simulink model "SOH_RLS_estimator_prev"  (R2024a)
settings: configuration reference "BMS_Base_ModelReferencingConfig" (kept outside this file)
values from neighbouring files (symbols this model uses):
  BATTERY_MODULE_CAPACITY_AH = 51.0    [ParametersDataDictionary.sldd]    (also in SOXDictionary.sldd; SOXDictionaryGotion.sldd = 116.0
  SOH_DOD_THRESHOLD = 0.1    [SOXDictionary.sldd]    (also in SOXDictionaryGotion.sldd = 0.1
  SOH_ESTIM_INIT = 1.0    [SOXDictionary.sldd]    (also in SOXDictionaryGotion.sldd = 1.0
  SOH_INITIAL_COVARIANCE = 1.0    [SOXDictionary.sldd]    (also in SOXDictionaryGotion.sldd = 1.0
  SOH_LAMBDA = 0.9995    [SOXDictionary.sldd]    (also in SOXDictionaryGotion.sldd = 0.9995
  SOH_TIMESTEP = 1.0    [SOXDictionary.sldd]    (also in SOXDictionaryGotion.sldd = 1.0
  TOTAL_N_CELL_VOLTAGE = 24    [SOXDictionary.sldd]
settings Model: DataDictionary=BcuModel.sldd  SimulationMode=accelerator  Creator=mmackenzie  LastModifiedBy=jgavidia
settings ConfigSetRef: SourceName=BMS_Base_ModelReferencingConfig

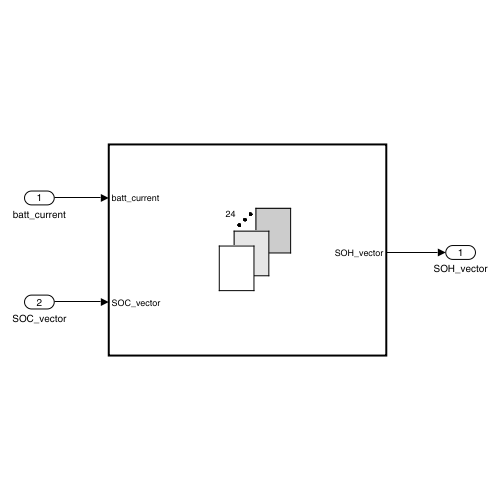
[thumbnail: Simulink's stored preview of the top-level diagram]
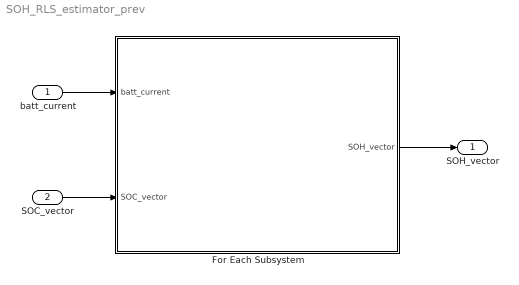
== system SOH_RLS_estimator_prev ==
  batt_current : Inport  OutDataTypeStr=int32  PortDimensions=1
  SOC_vector : Inport  Port=2  OutDataTypeStr=uint16  PortDimensions=[TOTAL_N_CELL_VOLTAGE,1]
  For Each Subsystem : Subsystem  TreatAsAtomicUnit=on
  SOH_vector : Outport  OutDataTypeStr=single  PortDimensions=[TOTAL_N_CELL_VOLTAGE,1]
  wires:
  batt_current/1 -> For Each Subsystem/1(batt_current)
  SOC_vector/1 -> For Each Subsystem/2(SOC_vector)
  For Each Subsystem/1(SOH_vector) -> SOH_vector/1

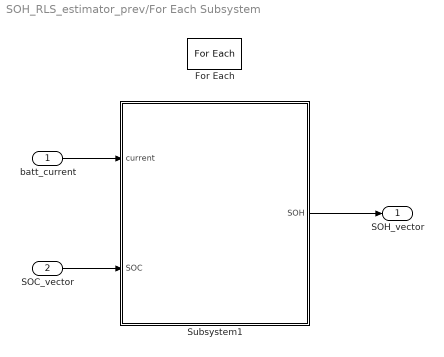
== system SOH_RLS_estimator_prev/For Each Subsystem ==
  batt_current : Inport  OutDataTypeStr=int32  PortDimensions=1
  SOC_vector : Inport  Port=2  OutDataTypeStr=uint16  PortDimensions=1  Partition=on  PartitionDimension=1  PartitionWidth=1  PartitionOffset=0
  For Each : ForEach  DisableCoverage=on
  Subsystem1 : Subsystem
  SOH_vector : Outport  OutDataTypeStr=single  PortDimensions=1  ConcatenationDimension=1
  wires:
  Subsystem1/1(SOH) -> SOH_vector/1
  batt_current/1 -> Subsystem1/1(current)
  SOC_vector/1 -> Subsystem1/2(SOC)

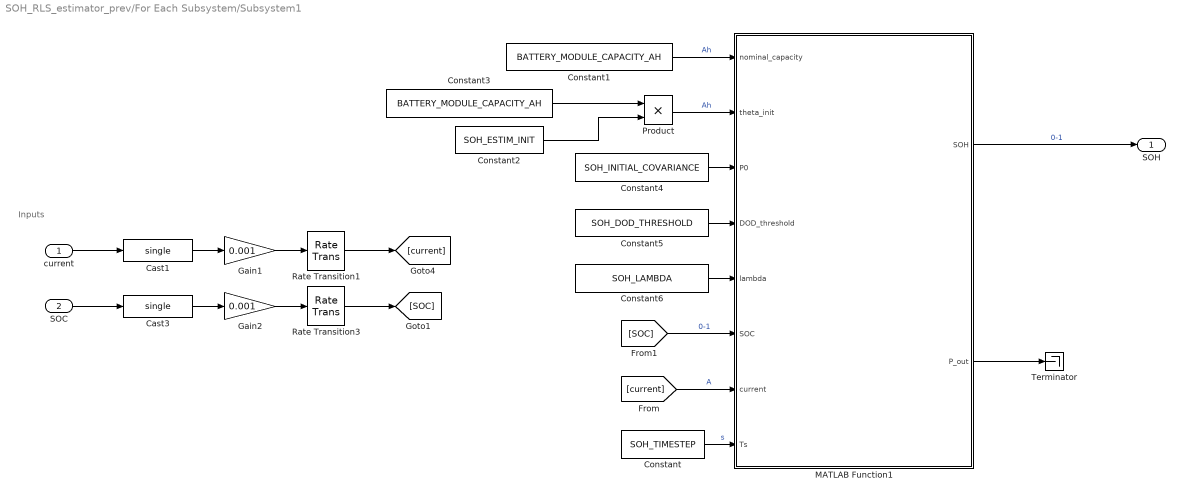
== system SOH_RLS_estimator_prev/For Each Subsystem/Subsystem1 ==
  note: Inputs
  current : Inport  OutDataTypeStr=int32  PortDimensions=1
  SOC : Inport  Port=2  OutDataTypeStr=uint16  PortDimensions=1
  Cast1 : DataTypeConversion  OutDataTypeStr=single  SaturateOnIntegerOverflow=off  RndMeth=Floor
  Cast3 : DataTypeConversion  OutDataTypeStr=single  SaturateOnIntegerOverflow=off  RndMeth=Floor
  Constant : Constant  Value=SOH_TIMESTEP
  Constant1 : Constant  Value=BATTERY_MODULE_CAPACITY_AH
  Constant2 : Constant  Value=SOH_ESTIM_INIT
  Constant3 : Constant  Value=BATTERY_MODULE_CAPACITY_AH
  Constant4 : Constant  Value=SOH_INITIAL_COVARIANCE
  Constant5 : Constant  Value=SOH_DOD_THRESHOLD
  Constant6 : Constant  Value=SOH_LAMBDA
  Gain1 : Gain  Gain=0.001
  Gain2 : Gain  Gain=0.001
  MATLAB Function1 : MATLAB Function  TreatAsAtomicUnit=on
  Product : Product
  Rate Transition1 : RateTransition  Integrity=off  OutPortSampleTime=1
  Rate Transition3 : RateTransition  Integrity=off  OutPortSampleTime=1
  Terminator : Terminator
  SOH : Outport  OutDataTypeStr=single  PortDimensions=1
  wires:
  Rate Transition1/1 -> [current]
  [SOC] -> MATLAB Function1/6(SOC)  "0-1"
  Constant1/1 -> MATLAB Function1/1(nominal_capacity)  "Ah"
  MATLAB Function1/2(P_out) -> Terminator/1
  Gain2/1 -> Rate Transition3/1
  Gain1/1 -> Rate Transition1/1
  [current] -> MATLAB Function1/7(current)  "A"
  Cast3/1 -> Gain2/1
  Rate Transition3/1 -> [SOC]
  current/1 -> Cast1/1
  Cast1/1 -> Gain1/1
  Constant/1 -> MATLAB Function1/8(Ts)  "s"
  SOC/1 -> Cast3/1
  MATLAB Function1/1(SOH) -> SOH/1  "0-1"
  Product/1 -> MATLAB Function1/2(theta_init)  "Ah"
  Constant3/1 -> Product/1
  Constant2/1 -> Product/2
  Constant4/1 -> MATLAB Function1/3(P0)
  Constant5/1 -> MATLAB Function1/4(DOD_threshold)
  Constant6/1 -> MATLAB Function1/5(lambda)

== matlab function SOH_RLS_estimator_prev/For Each Subsystem/Subsystem1/MATLAB Function1 ==
  data: nominal_capacity input; theta_init input; P0 input; DOD_threshold input; lambda input; SOH output; SOC input; current input; Ts input; P_out output
function [SOH, P_out] = SOH_Capacity_RLS(nominal_capacity, theta_init, P0, DOD_threshold, lambda, SOC, current, Ts)
    % nominal_capacity: Nominal capacity of the battery (Ah)
    % theta_init: Initial guess of the capacity (Ah)
    % SOC: 0 to 1
    % current: Current in A
    % Ts: Timestep (1s)

    lambda = single(lambda);
    
    % RLS memory
    persistent theta P accum_Ah last_soc
    
    % --- 1. INITIALIZATION ---
    if isempty(theta)
        theta = single(theta_init); % Initial guess
        P = single(P0);       % Initial uncertainty (large for faster initial learning)
        accum_Ah = single(0);  % Accumulator for Amp-hours
        last_soc = single(SOC);
    end

    % --- 2. DATA ACCUMULATION ---
    % Only accumulate if current is significant to avoid noise/offset
    if abs(current) > 0.05
        accum_Ah = accum_Ah + (current * Ts / 3600);
    end

    % Calculate the SOC swing since the last update
    delta_soc = SOC - last_soc;

    % --- 3. THE RLS UPDATE LOGIC ---
    % Update the Capacity estimate after a significant SOC swing (e.g., 10%).
    % Small swings are dominated by sensor noise and would cause SOH to jump.
    if abs(delta_soc) > DOD_threshold
        % RLS core: y = theta * x
        y = abs(accum_Ah);
        x = abs(delta_soc);
        
        % Prediction error
        error = y - (theta * x);
        
        % Calculate Gain for RLS
        K = (P * x) / (lambda + x * P * x);
        
        % Update the Capacity estimate (theta) and Covariance (P)
        theta = theta + K * error;
        P = (P - K * x * P) / lambda;
        
        % --- 4. HOUSEKEEPING ---
        % Reset the accumulators for the next "swing" segment
        accum_Ah = single(0);
        last_soc = SOC;
        
        % Safety Clamp: Capacity shouldn't exceed 110% or drop below 60% suddenly
        theta = max(0.6 * nominal_capacity, min(1.1 * nominal_capacity, theta));
    end

    % --- 5. OUTPUTS ---
    SOH = theta / nominal_capacity;
    P_out = P;
end
